simulink model "MAVDynamics"  (R2017b)
settings: Solver=ode4  StartTime=0.0  StopTime=20  FixedStep=sim_step  RelTol=1e-3  EnableMultiTasking=on
undefined symbols (not defined in the file): g, initlinvel, initpos, initRotMat, initrotvel, J, m
settings Model: Creator=Burak  LastModifiedBy=buyue
settings DataIOCC: LimitDataPoints=on  SaveFormat=Array
settings OptimizationCC: LifeSpan=inf
settings DebuggingCC: UnderspecifiedInitializationDetection=Classic  MergeDetectMultiDrivingBlocksExec=none  SolverPrmCheckMsg=warning  StateNameClashWarn=warning  SFUnexpectedBacktrackingDiag=warning  SFNoUnconditionalDefaultTransitionDiag=warning  SFExecutionAtInitializationDiag=none
settings HardwareCC: ProdBitPerPointer=32  ProdBitPerSizeT=32  ProdBitPerPtrDiffT=32  ProdLargestAtomicFloat=None  ProdIntDivRoundTo=Undefined  ProdEndianess=Unspecified  ProdWordSize=32  ProdHWDeviceType=32-bit Generic
settings ModelReferenceCC: PropagateSignalLabelsOutOfModel=off
settings CodeAppCC: StateflowObjectComments=on
settings GRTTargetCC: TargetLangStandard=C89/C90 (ANSI)  GeneratePreprocessorConditionals=Disable all
settings ConfigComp: CovMetricSettings=dw  CovHtmlReporting=on  CovSaveCumulativeToWorkspaceVar=on  CovSaveSingleToWorkspaceVar=on  CovExternalEMLEnable=off

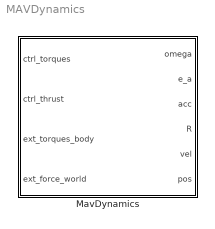
== system MAVDynamics ==
  MavDynamics : Subsystem

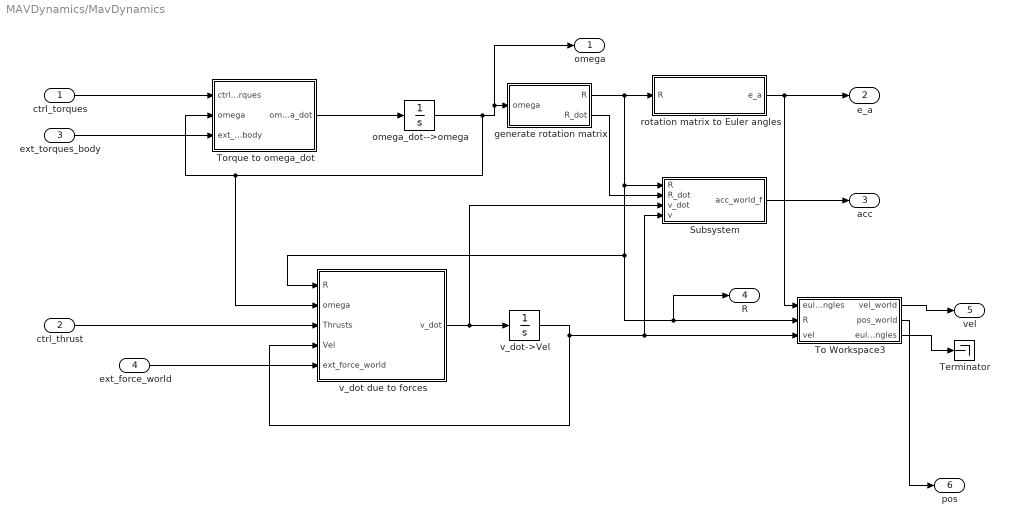
== system MAVDynamics/MavDynamics ==
  ctrl_torques : Inport
  ctrl_thrust : Inport  Port=2
  ext_torques_body : Inport  Port=3
  ext_force_world : Inport  Port=4
  Subsystem : Subsystem
  Terminator : Terminator
  To Workspace3 : Subsystem
  Torque to omega_dot : Subsystem
  generate rotation matrix : Subsystem
  omega_dot-->omega : Integrator  InitialCondition=initrotvel
  rotation matrix to Euler angles : MATLAB Function  TreatAsAtomicUnit=on
  v_dot due to forces : Subsystem
  v_dot->Vel : Integrator  InitialCondition=initlinvel
  omega : Outport
  e_a : Outport  Port=2
  acc : Outport  Port=3
  R : Outport  Port=4
  vel : Outport  Port=5
  pos : Outport  Port=6
  wires:
  To Workspace3/3("euler_angles ") -> Terminator/1
  v_dot due to forces/1(v_dot) -> Subsystem/3(v_dot), v_dot->Vel/1
  omega_dot-->omega/1 -> v_dot due to forces/2(omega), Torque to omega_dot/2(omega), omega/1, generate rotation matrix/1(omega)
  ext_force_world/1 -> v_dot due to forces/5(ext_force_world)
  To Workspace3/2(pos_world) -> pos/1
  Subsystem/1(acc_world_f) -> acc/1
  To Workspace3/1(vel_world) -> vel/1
  ctrl_thrust/1 -> v_dot due to forces/3(Thrusts)
  rotation matrix to Euler angles/1(e_a) -> e_a/1, To Workspace3/1(euler_angles)
  ext_torques_body/1 -> Torque to omega_dot/3(ext_torques_body)
  Torque to omega_dot/1(omega_dot) -> omega_dot-->omega/1
  generate rotation matrix/1(R) -> rotation matrix to Euler angles/1(R), R/1, To Workspace3/2(R), v_dot due to forces/1(R), Subsystem/1(R)
  v_dot->Vel/1 -> To Workspace3/3(vel), Subsystem/4(v), v_dot due to forces/4(Vel)
  generate rotation matrix/2(R_dot) -> Subsystem/2(R_dot)
  ctrl_torques/1 -> Torque to omega_dot/1(ctrl_orques)

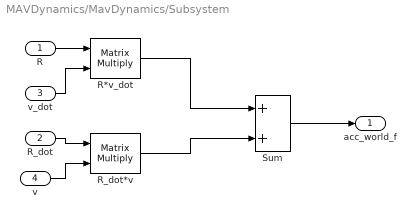
== system MAVDynamics/MavDynamics/Subsystem ==
  R : Inport
  R_dot : Inport  Port=2
  v_dot : Inport  Port=3
  v : Inport  Port=4
  R*v_dot : Product  Multiplication=Matrix(*)  RndMeth=Zero
  R_dot*v : Product  Multiplication=Matrix(*)  RndMeth=Zero
  Sum : Sum
  acc_world_f : Outport
  wires:
  Sum/1 -> acc_world_f/1
  R/1 -> R*v_dot/1
  v_dot/1 -> R*v_dot/2
  R_dot/1 -> R_dot*v/1
  v/1 -> R_dot*v/2
  R*v_dot/1 -> Sum/1
  R_dot*v/1 -> Sum/2

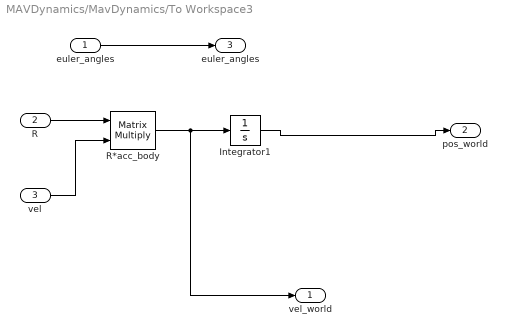
== system MAVDynamics/MavDynamics/To Workspace3 ==
  euler_angles : Inport
  R : Inport  Port=2
  vel : Inport  Port=3
  Integrator1 : Integrator  InitialCondition=initpos
  R*acc_body : Product  Multiplication=Matrix(*)  RndMeth=Zero
  vel_world : Outport
  pos_world : Outport  Port=2
  "euler_angles " : Outport  Port=3
  wires:
  R/1 -> R*acc_body/1
  vel/1 -> R*acc_body/2
  euler_angles/1 -> "euler_angles "/1
  R*acc_body/1 -> vel_world/1, Integrator1/1
  Integrator1/1 -> pos_world/1

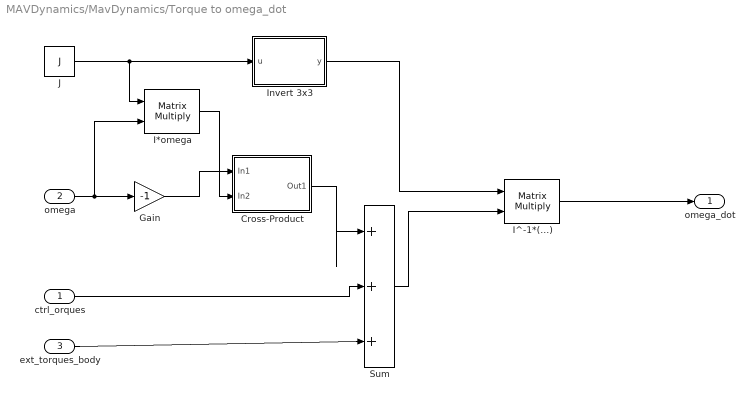
== system MAVDynamics/MavDynamics/Torque to omega_dot ==
  ctrl_orques : Inport
  omega : Inport  Port=2
  ext_torques_body : Inport  Port=3
  Cross-Product : Subsystem
  Gain : Gain  Gain=-1
  I*omega : Product  Multiplication=Matrix(*)  RndMeth=Zero
  I^-1*(...) : Product  Multiplication=Matrix(*)  RndMeth=Zero
  Invert 3x3 : MATLAB Function  TreatAsAtomicUnit=on
  J : Constant  Value=J
  Sum : Sum  Inputs=|+++
  omega_dot : Outport
  wires:
  omega/1 -> I*omega/2, Gain/1
  J/1 -> I*omega/1, Invert 3x3/1(u)
  I*omega/1 -> Cross-Product/2(In2)
  Invert 3x3/1(y) -> I^-1*(...)/1
  I^-1*(...)/1 -> omega_dot/1
  ctrl_orques/1 -> Sum/2
  Sum/1 -> I^-1*(...)/2
  Gain/1 -> Cross-Product/1(In1)
  Cross-Product/1(Out1) -> Sum/1
  ext_torques_body/1 -> Sum/3

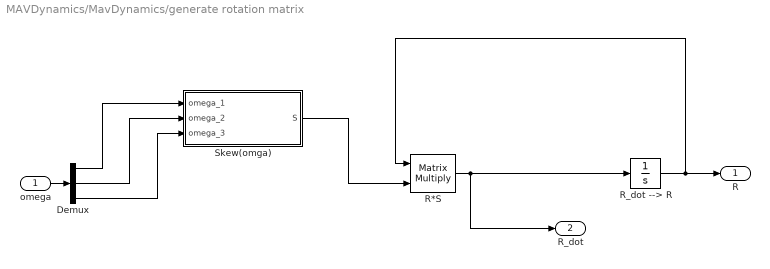
== system MAVDynamics/MavDynamics/generate rotation matrix ==
  omega : Inport
  Demux : Demux  Outputs=3
  R*S : Product  Multiplication=Matrix(*)  RndMeth=Zero
  R_dot --> R : Integrator  InitialCondition=initRotMat
  Skew(omga) : MATLAB Function  TreatAsAtomicUnit=on
  R : Outport
  R_dot : Outport  Port=2
  wires:
  R*S/1 -> R_dot --> R/1, R_dot/1
  R_dot --> R/1 -> R/1, R*S/1
  omega/1 -> Demux/1
  Demux/1 -> Skew(omga)/1(omega_1)
  Demux/2 -> Skew(omga)/2(omega_2)
  Demux/3 -> Skew(omga)/3(omega_3)
  Skew(omga)/1(S) -> R*S/2

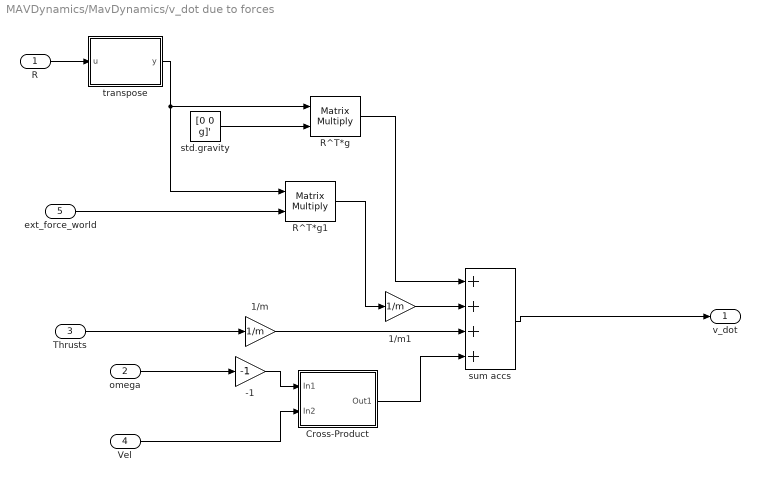
== system MAVDynamics/MavDynamics/v_dot due to forces ==
  R : Inport
  omega : Inport  Port=2
  Thrusts : Inport  Port=3
  Vel : Inport  Port=4
  ext_force_world : Inport  Port=5
  -1 : Gain  Gain=-1
  1/m : Gain  Gain=1/m
  1/m1 : Gain  Gain=1/m
  Cross-Product : Subsystem
  R^T*g : Product  Multiplication=Matrix(*)  RndMeth=Zero
  R^T*g1 : Product  Multiplication=Matrix(*)  RndMeth=Zero
  std.gravity : Constant  Value=[0 0 g]'
  sum accs : Sum  Inputs=++++
  transpose : MATLAB Function  TreatAsAtomicUnit=on
  v_dot : Outport
  wires:
  omega/1 -> -1/1
  Vel/1 -> Cross-Product/2(In2)
  R/1 -> transpose/1(u)
  transpose/1(y) -> R^T*g1/1, R^T*g/1
  std.gravity/1 -> R^T*g/2
  R^T*g/1 -> sum accs/1
  sum accs/1 -> v_dot/1
  Thrusts/1 -> 1/m/1
  -1/1 -> Cross-Product/1(In1)
  Cross-Product/1(Out1) -> sum accs/4
  1/m/1 -> sum accs/3
  ext_force_world/1 -> R^T*g1/2
  R^T*g1/1 -> 1/m1/1
  1/m1/1 -> sum accs/2

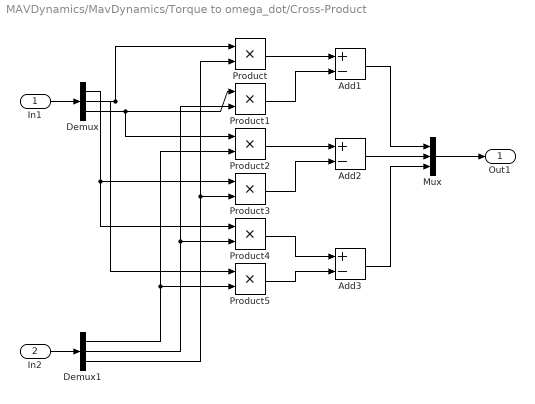
== system MAVDynamics/MavDynamics/Torque to omega_dot/Cross-Product ==
  In1 : Inport
  In2 : Inport  Port=2
  Add1 : Sum  Inputs=+-
  Add2 : Sum  Inputs=+-
  Add3 : Sum  Inputs=+-
  Demux : Demux  Outputs=3
  Demux1 : Demux  Outputs=3
  Mux : Mux  Inputs=3
  Product{,1..5} (6 alike) : Product  RndMeth=Zero
  Out1 : Outport
  wires:
  In1/1 -> Demux/1
  In2/1 -> Demux1/1
  Mux/1 -> Out1/1
  Add1/1 -> Mux/1
  Add2/1 -> Mux/2
  Add3/1 -> Mux/3
  Demux/2 -> Product/1, Product5/1
  Demux1/3 -> Product/2, Product3/2
  Demux/3 -> Product1/1, Product2/1
  Demux1/2 -> Product1/2, Product4/2
  Demux/1 -> Product3/1, Product4/1
  Demux1/1 -> Product2/2, Product5/2
  Product/1 -> Add1/1
  Product1/1 -> Add1/2
  Product2/1 -> Add2/1
  Product3/1 -> Add2/2
  Product4/1 -> Add3/1
  Product5/1 -> Add3/2

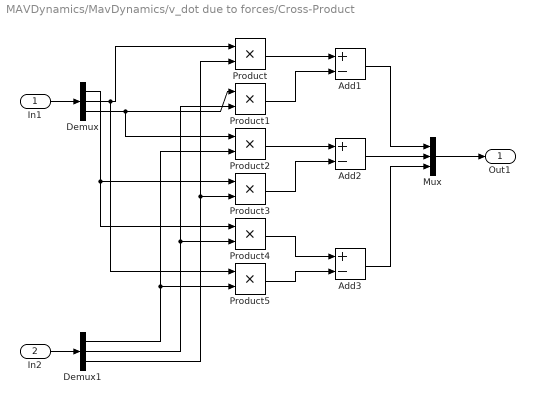
== system MAVDynamics/MavDynamics/v_dot due to forces/Cross-Product ==
  In1 : Inport
  In2 : Inport  Port=2
  Add1 : Sum  Inputs=+-
  Add2 : Sum  Inputs=+-
  Add3 : Sum  Inputs=+-
  Demux : Demux  Outputs=3
  Demux1 : Demux  Outputs=3
  Mux : Mux  Inputs=3
  Product{,1..5} (6 alike) : Product  RndMeth=Zero
  Out1 : Outport
  wires:
  In1/1 -> Demux/1
  In2/1 -> Demux1/1
  Mux/1 -> Out1/1
  Add1/1 -> Mux/1
  Add2/1 -> Mux/2
  Add3/1 -> Mux/3
  Demux/2 -> Product/1, Product5/1
  Demux1/3 -> Product/2, Product3/2
  Demux/3 -> Product1/1, Product2/1
  Demux1/2 -> Product1/2, Product4/2
  Demux/1 -> Product3/1, Product4/1
  Demux1/1 -> Product2/2, Product5/2
  Product/1 -> Add1/1
  Product1/1 -> Add1/2
  Product2/1 -> Add2/1
  Product3/1 -> Add2/2
  Product4/1 -> Add3/1
  Product5/1 -> Add3/2

== matlab function MAVDynamics/MavDynamics/Torque to omega_dot/Invert 3x3 ==
  data: u input; y output
function y = fcn(u)


y = NaN(3,3);
y(1,1) = u(3,3)*u(2,2)- u(2,3)*u(3,2);
y(1,2) = u(1,3)*u(3,2)- u(3,3)*u(1,2);
y(1,3) = u(1,2)*u(2,3)- u(2,2)*u(1,3);

y(2,1) = u(2,3)*u(3,1)- u(2,1)*u(3,3);
y(2,2) = u(1,1)*u(3,3)- u(3,1)*u(1,3);
y(2,3) = u(1,3)*u(2,1)- u(1,1)*u(2,3);

y(3,1) = u(2,1)*u(3,2)- u(2,2)*u(3,1);
y(3,2) = u(1,2)*u(3,1)- u(1,1)*u(3,2);
y(3,3) = u(1,1)*u(2,2)- u(1,2)*u(2,1);

y=1/det(u)*y;

== matlab function MAVDynamics/MavDynamics/generate rotation matrix/Skew(omga) ==
  data: omega_1 input; S output; omega_2 input; omega_3 input
function S = skew(omega_1, omega_2, omega_3)
% This block supports the Embedded MATLAB subset.
% See the help menu for details. 
S = [0 -omega_3 omega_2;
 omega_3 0 -omega_1;
 -omega_2 omega_1 0];

== matlab function MAVDynamics/MavDynamics/rotation matrix to Euler angles ==
  data: R input; e_a output
function e_a = eulerangles(R)
% This block supports an embeddable subset of the MATLAB language.
% See the help menu for details. 

e_a = zeros(3,1);

Roll = atan2(R(3,2),R(3,3));
Pitch = atan2(-R(3,1),sqrt(R(3,2)^2+R(3,3)^2));
Yaw = atan2(R(2,1),R(1,1));


e_a = [Roll; Pitch; Yaw];

== matlab function MAVDynamics/MavDynamics/v_dot due to forces/transpose ==
  data: u input; y output
function y = fcn(u)
% This block supports the Embedded MATLAB subset.
% See the help menu for details. 

y = u';
